simulink model "Experiment_0309_cs_old"  (R2019a)
settings: Solver=ode5  StartTime=0.0  StopTime=6  FixedStep=1/120  RelTol=1e-3
PreLoadFcn:
  | mbxruntime.callbacks.PreLoadFcn(bdroot);
PostLoadFcn:
  | mbxruntime.callbacks.PostLoadFcn(bdroot);
InitFcn:
  | mbxruntime.callbacks.InitFcn(bdroot);
StartFcn:
  | mbxruntime.callbacks.StartFcn(bdroot);
StopFcn:
  | mbxruntime.callbacks.StopFcn(bdroot);
model workspace (MAT data in the model file):
  mbox_table : struct (value not decoded)
  model_closed = 0
  sim_status = 0
undefined symbols (not defined in the file or in its folder): DiscIntNeverNeededParam, InitImageOutputDir, mbxruntime, tabledata
libraries: PreScanSimulinkLibrary x24, simulink_extras x2
(part 1 of 3)
CloseFcn:
  | mbxruntime.callbacks.CloseFcn(bdroot);
settings Model: Creator=PRESCAN  LastModifiedBy=HP
settings DataIOCC: LimitDataPoints=on  SaveFormat=Array  SignalLoggingSaveFormat=ModelDataLogs  ReturnWorkspaceOutputs=off
settings OptimizationCC: ExpressionDepthLimit=2147483647  InitFltsAndDblsToZero=on  LifeSpan=inf
settings DebuggingCC: SaveWithParameterizedLinksMsg=none  UnderspecifiedInitializationDetection=Classic  MergeDetectMultiDrivingBlocksExec=none  SignalResolutionControl=TryResolveAllWithWarning  MultiTaskDSMMsg=warning  MultiTaskCondExecSysMsg=none  FcnCallInpInsideContextMsg=warning  StateNameClashWarn=warning  SFUnexpectedBacktrackingDiag=warning  SFNoUnconditionalDefaultTransitionDiag=warning  SFExecutionAtInitializationDiag=none  ArithmeticOperatorsInVariantConditions=warning
settings HardwareCC: ProdBitPerPointer=32  ProdBitPerSizeT=32  ProdBitPerPtrDiffT=32  ProdLargestAtomicFloat=None  ProdIntDivRoundTo=Undefined  ProdEndianess=Unspecified  ProdWordSize=32  ProdHWDeviceType=32-bit Generic
settings ModelReferenceCC: UpdateModelReferenceTargets=IfOutOfDate  PropagateSignalLabelsOutOfModel=off
settings SFSimCC: SimUseLocalCustomCode=off  SimParseCustomCode=off
settings SFSimCC: SimCustomHeaderCode=|
  | #include "prescan.h"
  | #include "prescan_platform.h"
settings RTWCC: RTWUseLocalCustomCode=off
settings CodeAppCC: StateflowObjectComments=on
settings GRTTargetCC: TargetFcnLib=ansi_tfl_tmw.mat  TargetLangStandard=C89/C90 (ANSI)  GeneratePreprocessorConditionals=Disable all  CombineOutputUpdateFcns=off  GRTInterface=on
settings ConfigComp: CovMetricSettings=dw  CovHtmlReporting=on  CovSaveCumulativeToWorkspaceVar=on  CovSaveSingleToWorkspaceVar=on  CovExternalEMLEnable=off

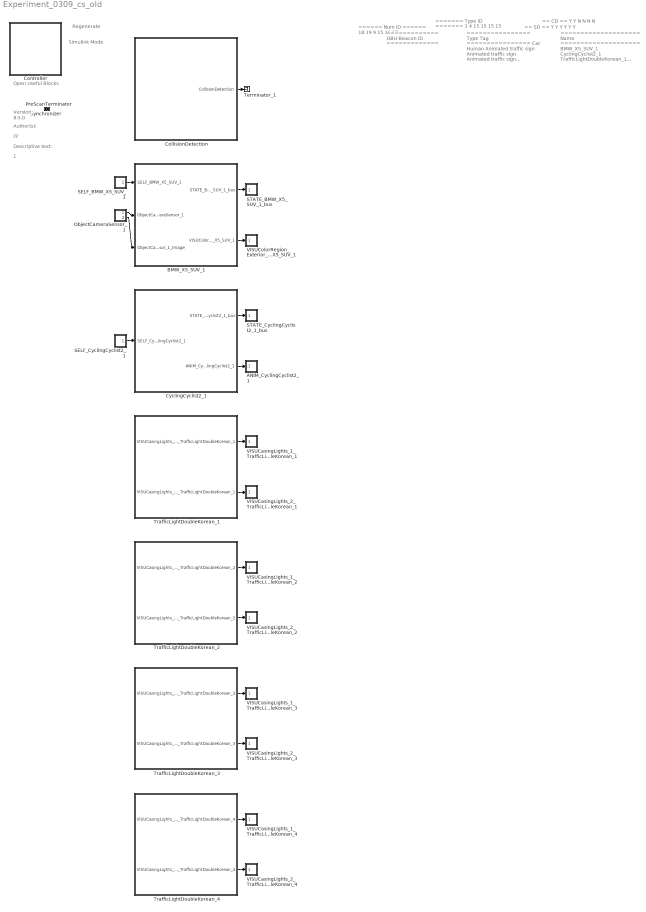
== system Experiment_0309_cs_old ==
  note: Regenerate
  note: Simulink Mode
  note: Open Useful Blocks
  note: 8.5.0
  note: Version:
  note: Author(s):
  note: zz
  note: Descriptive text:
  note: 1
  note: ======
      | Num ID
      | ======
      | 18
      | 19
      | 9
      | 15
      | 16
      | 17
  note: =============
      | OBU-Beacon ID
      | =============
  note: =======
      | Type ID
      | =======
      | 1
      | 4
      | 15
      | 15
      | 15
      | 15
  note: ================
      | Type Tag
      | ================
      | Car
      | Human
      | Animated traffic sign
      | Animated traffic sign
      | Animated traffic sign
      | Animated traffic sign
  note: ==
      | SD
      | ==
      | Y
      | Y
      | Y
      | Y
      | Y
      | Y
  note: ==
      | CD
      | ==
      | Y
      | Y
      | N
      | N
      | N
      | N
  note: ====================
      | Name
      | ====================
      | BMW_X5_SUV_1
      | CyclingCyclist2_1
      | TrafficLightDoubleKorean_1
      | TrafficLightDoubleKorean_2
      | TrafficLightDoubleKorean_3
      | TrafficLightDoubleKorean_4
  ANIM_CyclingCyclist2_1 : Subsystem  Tag=actuator/AnimationOutport  Priority=0  LoadFcn=load('PreScanAnimActuatorData.mat')  mask(PreScan Sink Block: State Animation){}
      mask help: The Cyclist Animation port allows the cyclist to ride the bicycle.
      settings: OpenFcn=open_system([gcb '/Actuator'],'mask')
      mask Help: eval('openHelp(239)')
      mask Display: image(imread('CyclingCyclist2.jpg'))
  BMW_X5_SUV_1 : Subsystem  Tag=WorldObjectSubSystem  InitFcn=UniqueId = '266';
      mask init:
      | modelPath = GenericModelHelper.getGenericModelFilePath('ModelDepo','Vehicles\BMW_X5\BMW_X5.pgmb','cea918691563e9ae3e6a88ec95e6726a');imagePath = GenericModelHelper.getCompilationPicture(modelPath, 'BMW_X5_HighPoly.png');
      mask Display: image(imread(imagePath));color('white');text(0, 0, ' ID=18\n')
  CollisionDetection : Subsystem  Tag=sensor/CollisionDetection  Priority=3  LoadFcn=load('PrescanCollisionDetectionData.mat');load('PrescanCollisionDetectionMessage.mat')  mask(PreScan Source Block: CollisionDetection){}
      mask help: Collision Detection can be used to detect collisions between PreScan components. For Collision Detection the actual component shape is taken into account, so it is not a bounding box approach.
      settings: OpenFcn=open_system([gcb '/Sensor'],'mask')
      mask Help: eval('openHelp(811)')
      mask Display: image(imread('crash.jpg'))
  Controller : Subsystem  Description=44ADF3809AA2EBDEE5B0ED277FCD47A88214DB959FC05F626C23B16B15099040  Priority=-1  LoadFcn=load PreScanControllerData  mask(PreScan Simulation Controller){prescanversion='8.5.0', ModelReferencing=off, TimeStep=3/120, ControlMode=0, PreScanExecutionMode=on, ControllerCount=0, ControllerIndex=0, ControllerOptions=''}
      mask prompts: prescanversion "PreScan Version"; ModelReferencing "Use Model Referencing"; TimeStep "Upload Period [s]"; ControlMode "Control Mode"; PreScanExecutionMode "Execution Mode"; ControllerCount "Controller Count"; ControllerIndex "Controller Index"; ControllerOptions "Controller Options"
      mask help:
      | Please do not remove this block from the compilation sheet,
      | as it connects the model to the PreScan environment.
      mask init:
      | model = bdroot(gcb);
      | ExperimentFile = mbxruntime.findExperimentFile(model,true); %relative path
      | 
      | [d1, d2, d3, prescandata] = prescan_Settings();
      | ModelDepo = fullfile(prescandata,'ModelDepo'); 
      | 
      | RTmode = mbxruntime.getRTMode(model);
      | 
      | SimulationMode = get_param(bdroot,'SimulationMode');
      | if strcmp(SimulationMode, 'rapid-accelerator')
      |     SimulationMode = 'external';
      | end
      | TargetName = get_param(bdroot,'SystemTargetFile');
      settings: ModelCloseFcn=assignin('base',['model_closed_' bdroot],true);
      mask Help: eval('openHelp(812)')
      mask Display: image(imread('prescanlogo.ico'))
  CyclingCyclist2_1 : Subsystem  Tag=WorldObjectSubSystem  InitFcn=UniqueId = '309';
      mask init:
      | imagePath=which('CyclingCyclist2.jpg');
      mask Display: image(imread(imagePath));color('white');text(0, 0, ' ID=19\n')
  ObjectCameraSensor_1 : Subsystem  Tag=sensor/ObjectCamera/data  Priority=3  LoadFcn=load('PrescanOCSData.mat');load('PrescanOCSMessage.mat')  mask(PreScan Source Block: Object Camera Sensor){}
      mask help: The Object Camera Sensor provides information on objects locations.
      settings: OpenFcn=open_system([gcb '/Sensor'],'mask')
      mask Help: eval('openHelp(2401)')
      mask Display: image(imread('ObjectCameraSensorSL.png'))
  PreScanTerminator : Subsystem  Tag=PreScanTerminator  Priority=999  LoadFcn=load PrescanTerminatorData  mask(PreScan Simulation Terminator){TimeStep=3/120}
      mask prompts: TimeStep "Upload Period [s]"
      mask help:
      | Please do not remove this block from the compilation sheet as it
      | connects the model to the PreScan environment.
      mask Help: eval('openHelp(812)')
      mask Display: image(imread('prescanlogo.ico'))
  SELF_BMW_X5_SUV_1 : Subsystem  Tag=sensor/SelfPort  Priority=3  LoadFcn=load('PreScanSelfSensorData.mat')  mask(PreScan Source Block: SELF){}
      mask help:
      | The SELF port shows (state) information of the actor itself. The outputs are position in the experiment's axis system and the GPS coordinates, and the object's absolute velocity and compass heading.
      |
      | For more information, please click Help.
      settings: OpenFcn=open_system([gcb '/Sensor'],'mask')
      mask Help: eval('openHelp(462)')
      mask Display: image(imread('GPS.png'))
  SELF_CyclingCyclist2_1 : Subsystem  Tag=sensor/SelfPort  Priority=3  LoadFcn=load('PreScanSelfSensorData.mat')  mask(PreScan Source Block: SELF){}
      mask help:
      | The SELF port shows (state) information of the actor itself. The outputs are position in the experiment's axis system and the GPS coordinates, and the object's absolute velocity and compass heading.
      |
      | For more information, please click Help.
      settings: OpenFcn=open_system([gcb '/Sensor'],'mask')
      mask Help: eval('openHelp(462)')
      mask Display: image(imread('GPS.png'))
  STATE_BMW_X5_SUV_1_bus : Subsystem  Tag=actuator/StatePort  Priority=0  LoadFcn=load('PreScanStateActuatorData.mat')  mask(PreScan Sink Block: State){}
      mask help:
      | The Actor State contains a vector signal of size (9x1), containing the following signals:
      |
      | -  Position    	(x,y,z)             	[m]
      | -  Velocity    	(vx,vy,vz)         	[m/s]
      | -  Angles       	(Roll, Pitch, Yaw)	[rad]
      |
      | The Actor state is defined in the global axis system.
      | The state is superponed on the Initial position defined in the GUI.
      |
      | For more information, please click Help.
      settings: OpenFcn=open_system([gcb '/Actuator'],'mask')
      mask Help: eval('openHelp(222)')
      mask Display: image(imread('State.png'))
  STATE_CyclingCyclist2_1_bus : Subsystem  Tag=actuator/StatePort  Priority=0  LoadFcn=load('PreScanStateActuatorData.mat')  mask(PreScan Sink Block: State){}
      mask help:
      | The Actor State contains a vector signal of size (9x1), containing the following signals:
      |
      | -  Position    	(x,y,z)             	[m]
      | -  Velocity    	(vx,vy,vz)         	[m/s]
      | -  Angles       	(Roll, Pitch, Yaw)	[rad]
      |
      | The Actor state is defined in the global axis system.
      | The state is superponed on the Initial position defined in the GUI.
      |
      | For more information, please click Help.
      settings: OpenFcn=open_system([gcb '/Actuator'],'mask')
      mask Help: eval('openHelp(222)')
      mask Display: image(imread('State.png'))
  Synchronizer : Subsystem  Tag=PreScanSynchronizer  Priority=1  LoadFcn=load PrescanSynchronizeData  mask(PreScan Simulation Core Block){TimeStep=3/120}
      mask prompts: TimeStep "Timestep [s]"
      mask help:
      | Please do not remove this block from the PreScan compilation sheet,
      | as it contains essential configuration parameters for a PreScan simulation.
      settings: DeleteFcn=PreScanBlockDeleteFcn;
      mask Display: image(imread('prescanlogo.ico'))
  Terminator_1 : Terminator
  TrafficLightDoubleKorean_1 : Subsystem  Tag=WorldObjectSubSystem  InitFcn=UniqueId = '262';
      mask init:
      | imagePath=which('TrafficLightDoubleKorean.jpg');
      mask Display: image(imread(imagePath));color('white');text(0, 0, ' ID=9\n')
  TrafficLightDoubleKorean_2 : Subsystem  Tag=WorldObjectSubSystem  InitFcn=UniqueId = '263';
      mask init:
      | imagePath=which('TrafficLightDoubleKorean.jpg');
      mask Display: image(imread(imagePath));color('white');text(0, 0, ' ID=15\n')
  TrafficLightDoubleKorean_3 : Subsystem  Tag=WorldObjectSubSystem  InitFcn=UniqueId = '264';
      mask init:
      | imagePath=which('TrafficLightDoubleKorean.jpg');
      mask Display: image(imread(imagePath));color('white');text(0, 0, ' ID=16\n')
  TrafficLightDoubleKorean_4 : Subsystem  Tag=WorldObjectSubSystem  InitFcn=UniqueId = '265';
      mask init:
      | imagePath=which('TrafficLightDoubleKorean.jpg');
      mask Display: image(imread(imagePath));color('white');text(0, 0, ' ID=17\n')
  VISUCasingLights_1_TrafficLightDoubleKorean_1 : Subsystem  Tag=actuator/VisuCasingLights  Priority=0  mask(PreScan Sink Block: VisuTrafficLight){UniqueID=262, ColorsObjectQuery=, Colors=[]}
      mask prompts: UniqueID "Parent Unique Identifier"; ColorsObjectQuery "Query for Color Object"; Colors "Matrix of colors"
      mask help:
      | The VisuTrafficLight block provides a way to animate traffic lights: switch on and off individual lights.
      |
      | For more information, please click Help.
      settings: OpenFcn=open_system([gcb '/Actuator'],'mask')
      mask Help: eval('openHelp(731)')
      mask Display: image(imread('TrafficLightCasing.png'))
  VISUCasingLights_1_TrafficLightDoubleKorean_2 : Subsystem  Tag=actuator/VisuCasingLights  Priority=0  mask(PreScan Sink Block: VisuTrafficLight){UniqueID=263, ColorsObjectQuery=, Colors=[]}
      mask prompts: UniqueID "Parent Unique Identifier"; ColorsObjectQuery "Query for Color Object"; Colors "Matrix of colors"
      mask help:
      | The VisuTrafficLight block provides a way to animate traffic lights: switch on and off individual lights.
      |
      | For more information, please click Help.
      settings: OpenFcn=open_system([gcb '/Actuator'],'mask')
      mask Help: eval('openHelp(731)')
      mask Display: image(imread('TrafficLightCasing.png'))
  VISUCasingLights_1_TrafficLightDoubleKorean_3 : Subsystem  Tag=actuator/VisuCasingLights  Priority=0  mask(PreScan Sink Block: VisuTrafficLight){UniqueID=264, ColorsObjectQuery=, Colors=[]}
      mask prompts: UniqueID "Parent Unique Identifier"; ColorsObjectQuery "Query for Color Object"; Colors "Matrix of colors"
      mask help:
      | The VisuTrafficLight block provides a way to animate traffic lights: switch on and off individual lights.
      |
      | For more information, please click Help.
      settings: OpenFcn=open_system([gcb '/Actuator'],'mask')
      mask Help: eval('openHelp(731)')
      mask Display: image(imread('TrafficLightCasing.png'))
  VISUCasingLights_1_TrafficLightDoubleKorean_4 : Subsystem  Tag=actuator/VisuCasingLights  Priority=0  mask(PreScan Sink Block: VisuTrafficLight){UniqueID=265, ColorsObjectQuery=, Colors=[]}
      mask prompts: UniqueID "Parent Unique Identifier"; ColorsObjectQuery "Query for Color Object"; Colors "Matrix of colors"
      mask help:
      | The VisuTrafficLight block provides a way to animate traffic lights: switch on and off individual lights.
      |
      | For more information, please click Help.
      settings: OpenFcn=open_system([gcb '/Actuator'],'mask')
      mask Help: eval('openHelp(731)')
      mask Display: image(imread('TrafficLightCasing.png'))
  VISUCasingLights_2_TrafficLightDoubleKorean_1 : Subsystem  Tag=actuator/VisuCasingLights  Priority=0  mask(PreScan Sink Block: VisuTrafficLight){UniqueID=262, ColorsObjectQuery=, Colors=[]}
      mask prompts: UniqueID "Parent Unique Identifier"; ColorsObjectQuery "Query for Color Object"; Colors "Matrix of colors"
      mask help:
      | The VisuTrafficLight block provides a way to animate traffic lights: switch on and off individual lights.
      |
      | For more information, please click Help.
      settings: OpenFcn=open_system([gcb '/Actuator'],'mask')
      mask Help: eval('openHelp(731)')
      mask Display: image(imread('TrafficLightCasing.png'))
  VISUCasingLights_2_TrafficLightDoubleKorean_2 : Subsystem  Tag=actuator/VisuCasingLights  Priority=0  mask(PreScan Sink Block: VisuTrafficLight){UniqueID=263, ColorsObjectQuery=, Colors=[]}
      mask prompts: UniqueID "Parent Unique Identifier"; ColorsObjectQuery "Query for Color Object"; Colors "Matrix of colors"
      mask help:
      | The VisuTrafficLight block provides a way to animate traffic lights: switch on and off individual lights.
      |
      | For more information, please click Help.
      settings: OpenFcn=open_system([gcb '/Actuator'],'mask')
      mask Help: eval('openHelp(731)')
      mask Display: image(imread('TrafficLightCasing.png'))
  VISUCasingLights_2_TrafficLightDoubleKorean_3 : Subsystem  Tag=actuator/VisuCasingLights  Priority=0  mask(PreScan Sink Block: VisuTrafficLight){UniqueID=264, ColorsObjectQuery=, Colors=[]}
      mask prompts: UniqueID "Parent Unique Identifier"; ColorsObjectQuery "Query for Color Object"; Colors "Matrix of colors"
      mask help:
      | The VisuTrafficLight block provides a way to animate traffic lights: switch on and off individual lights.
      |
      | For more information, please click Help.
      settings: OpenFcn=open_system([gcb '/Actuator'],'mask')
      mask Help: eval('openHelp(731)')
      mask Display: image(imread('TrafficLightCasing.png'))
  VISUCasingLights_2_TrafficLightDoubleKorean_4 : Subsystem  Tag=actuator/VisuCasingLights  Priority=0  mask(PreScan Sink Block: VisuTrafficLight){UniqueID=265, ColorsObjectQuery=, Colors=[]}
      mask prompts: UniqueID "Parent Unique Identifier"; ColorsObjectQuery "Query for Color Object"; Colors "Matrix of colors"
      mask help:
      | The VisuTrafficLight block provides a way to animate traffic lights: switch on and off individual lights.
      |
      | For more information, please click Help.
      settings: OpenFcn=open_system([gcb '/Actuator'],'mask')
      mask Help: eval('openHelp(731)')
      mask Display: image(imread('TrafficLightCasing.png'))
  VISUColorRegion_Exterior_BMW_X5_SUV_1 : Subsystem  Tag=actuator/ColorRegion  Priority=0  LoadFcn=load('PrescanColorData')  mask(PreScan Sink Block: VisuTextureColor){}
      mask help:
      | The VisuTextureColor block provides a way to adapt the color of a vehicle.
      |
      | For more information, please click Help.
      settings: OpenFcn=open_system([gcb '/Actuator'],'mask')
      mask Help: eval('openHelp(230)')
      mask Display: image(imread('TextureColor.png'))
  wires:
  BMW_X5_SUV_1/1(STATE_BMW_X5_SUV_1_bus) -> STATE_BMW_X5_SUV_1_bus/1(STATE_BMW_X5_SUV_1_bus)
  SELF_BMW_X5_SUV_1/1(SELF_BMW_X5_SUV_1) -> BMW_X5_SUV_1/1(SELF_BMW_X5_SUV_1)
  ObjectCameraSensor_1/1(ObjectCameraSensor_1) -> BMW_X5_SUV_1/2(ObjectCameraSensor_1)
  ObjectCameraSensor_1/2(ObjectCameraSensor_1_Image) -> BMW_X5_SUV_1/3(ObjectCameraSensor_1_Image)
  BMW_X5_SUV_1/2(VISUColorRegion_Exterior_BMW_X5_SUV_1) -> VISUColorRegion_Exterior_BMW_X5_SUV_1/1(VISUColorRegion_Exterior_BMW_X5_SUV_1)
  CyclingCyclist2_1/1(STATE_CyclingCyclist2_1_bus) -> STATE_CyclingCyclist2_1_bus/1(STATE_CyclingCyclist2_1_bus)
  CyclingCyclist2_1/2(ANIM_CyclingCyclist2_1) -> ANIM_CyclingCyclist2_1/1(ANIM_CyclingCyclist2_1)
  SELF_CyclingCyclist2_1/1(SELF_CyclingCyclist2_1) -> CyclingCyclist2_1/1(SELF_CyclingCyclist2_1)
  TrafficLightDoubleKorean_1/1(VISUCasingLights_1_TrafficLightDoubleKorean_1) -> VISUCasingLights_1_TrafficLightDoubleKorean_1/1(VISUCasingLights_1_TrafficLightDoubleKorean_1)
  TrafficLightDoubleKorean_1/2(VISUCasingLights_2_TrafficLightDoubleKorean_1) -> VISUCasingLights_2_TrafficLightDoubleKorean_1/1(VISUCasingLights_2_TrafficLightDoubleKorean_1)
  TrafficLightDoubleKorean_2/1(VISUCasingLights_1_TrafficLightDoubleKorean_2) -> VISUCasingLights_1_TrafficLightDoubleKorean_2/1(VISUCasingLights_1_TrafficLightDoubleKorean_2)
  TrafficLightDoubleKorean_2/2(VISUCasingLights_2_TrafficLightDoubleKorean_2) -> VISUCasingLights_2_TrafficLightDoubleKorean_2/1(VISUCasingLights_2_TrafficLightDoubleKorean_2)
  TrafficLightDoubleKorean_3/1(VISUCasingLights_1_TrafficLightDoubleKorean_3) -> VISUCasingLights_1_TrafficLightDoubleKorean_3/1(VISUCasingLights_1_TrafficLightDoubleKorean_3)
  TrafficLightDoubleKorean_3/2(VISUCasingLights_2_TrafficLightDoubleKorean_3) -> VISUCasingLights_2_TrafficLightDoubleKorean_3/1(VISUCasingLights_2_TrafficLightDoubleKorean_3)
  TrafficLightDoubleKorean_4/1(VISUCasingLights_1_TrafficLightDoubleKorean_4) -> VISUCasingLights_1_TrafficLightDoubleKorean_4/1(VISUCasingLights_1_TrafficLightDoubleKorean_4)
  TrafficLightDoubleKorean_4/2(VISUCasingLights_2_TrafficLightDoubleKorean_4) -> VISUCasingLights_2_TrafficLightDoubleKorean_4/1(VISUCasingLights_2_TrafficLightDoubleKorean_4)
  CollisionDetection/1(CollisionDetection) -> Terminator_1/1

== system Experiment_0309_cs_old/ANIM_CyclingCyclist2_1 ==
  ANIM_CyclingCyclist2_1 : Inport  Tag=inport/AnimationOutport  OutDataTypeStr=Bus: PRESCAN_ANIMACTUATORDATA  PortDimensions=2  SampleTime=3/120  BusOutputAsStruct=on
  Actuator : S-Function  FunctionName=sfun_CyclistAnimActuator  Parameters=UniqueID, uint8([ParentObject 0]), TimeStep  SFunctionDeploymentMode=off  EnableBusSupport=off  mask(PreScan Sink Block: State Animation){UniqueID=309, ParentObject=CyclingCyclist2_1, TimeStep=3/120}
      mask prompts: UniqueID "Auto-Assigned: Unique ID"; ParentObject "Auto-Assigned: ParentObject"; TimeStep "Auto-Assigned: Upload Period [s]"
      mask help: The Cyclist Animation port allows the cyclist to ride the bicycle.
      mask Help: eval('openHelp(239)')
      mask Display: image(imread('CyclingCyclist2.jpg'))
  wires:
  ANIM_CyclingCyclist2_1/1 -> Actuator/1

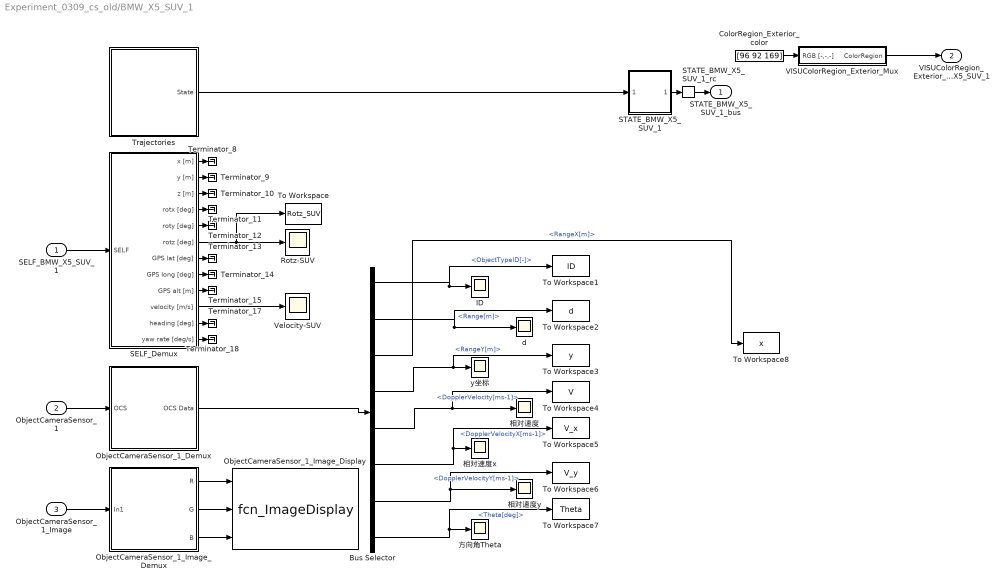
== system Experiment_0309_cs_old/BMW_X5_SUV_1 ==
  SELF_BMW_X5_SUV_1 : Inport  Tag=inport/SelfPort  OutDataTypeStr=Bus: PRESCAN_SELFSENSORDATA  PortDimensions=1  SampleTime=3/120  BusOutputAsStruct=on
  ObjectCameraSensor_1 : Inport  Tag=inport/ObjectCamera/data  Port=2  OutDataTypeStr=Bus: PRESCAN_OCS_MESSAGE  PortDimensions=7  SampleTime=1/40  BusOutputAsStruct=on
  ObjectCameraSensor_1_Image : Inport  Tag=inport/ObjectCamera/image  Port=3  OutDataTypeStr=uint8  SampleTime=1/40  BusOutputAsStruct=on
  Bus Selector : BusSelector  OutputSignals=ObjectTypeID[-],Range[m],RangeX[m],RangeY[m],DopplerVelocity[ms-1],DopplerVelocityX[ms-1],DopplerVelocityY[ms-1],Theta[deg]
  ColorRegion_Exterior_color : Constant  Tag=VisuLightConst  Value=[96 92 169]
  ID : Scope
  ObjectCameraSensor_1_Demux : Subsystem  Tag=demux/OCS  mask(PreScan Demux Block: Object Camera Sensor){detectableObjects=7}
      mask prompts: detectableObjects "Max. detectable objects"
      settings: DeleteFcn=PreScanBlockDeleteFcn;
      mask Help: eval('openHelp(2401)')
      mask Display:
      | port_label('input', 1, 'OCS')
      | port_label('output', 1, 'OCS Data')
  ObjectCameraSensor_1_Image_Demux : Subsystem  Tag=demux/Camera/Color  mask{SensorName=ObjectCameraSensor_1, hres=320, vres=240}
      mask prompts: SensorName "Sensor Name"; hres "Horizontal Resolution"; vres "Vertical Resolution"
      mask Help: eval('openHelp(2401)')
      mask Display:
      | fprintf('MONO CAMERA:\n Color\n %s \n %d x %d px',SensorName,hres,vres)
      | port_label('output',1,'R')
      | port_label('output',2,'G')
      | port_label('output',3,'B')
  ObjectCameraSensor_1_Image_Display : M-S-Function  Tag=CameraSensor_Color_Display  InitFcn=InitImageOutputDir(gcb);  FunctionName=fcn_ImageDisplay  Parameters=SensorName EnableDisplay EnablePosition DisplayPosition FigureHandle SaveResults BitmapFormat TempOutputDir CameraType DataType  mask(PreScan Color Display Block){SensorName=ObjectCameraSensor_1_Image, EnableDisplay=on, EnablePosition=off, DisplayPosition=[10 10 320 240], FigureHandle=26601, SaveResults=off, Format=PNG, TempOutputDir=0, CameraType=Mono, DataType=uint8}
      mask prompts: SensorName "User Specified: Title of Display"; EnableDisplay "Active"; EnablePosition "Set Display window position"; DisplayPosition "Display window position [xpos ypos width height]"; FigureHandle "Unique Handle"; SaveResults "Save results"; TempOutputDir "OutputDir"; CameraType "Camera Type"; DataType "Image Data Type"
      mask help: This block displays the RGB output of a PreScan camera sensor.
      mask init:
      | if EnableDisplay
      |     EnableString='';
      |     EnableColor='gray';
      | else
      |     EnableString='INACTIVE';
      |     EnableColor='red';
      | end
      | switch Format
      |     case 1
      |         BitmapFormat = 'png';
      |     case 2
      |         BitmapFormat = 'bmp';
      |     case 3
      |         BitmapFormat = 'jpg';
      | end 
      | if CameraType==1
      |     CameraTypeName='MONO';
      |     PortNumber=0;
      | else
      |     CameraTypeName='STEREO';
      |     PortNumber=3;
      | end
      settings: CopyFcn=CopyFcnDisplay  DeleteFcn=PreScanBlockDeleteFcn;  ModelCloseFcn=fcn_ImageDisplay_ModelCloseFcn
      mask Help: eval('openHelp(2401)')
      mask Callback EnablePosition:
      | MV=get_param(gcb,'MaskVisibilities');
      | if strcmp(get_param(gcb,'EnablePosition'),'on')
      |     MV{4}='on';
      | else
      |     MV{4}='off';
      | end
      | set_param(gcb,'MaskVisibilities',MV);
      | clear MV;
      mask TypeOptions Format: PNG | BMP | JPG
      mask TypeOptions CameraType: Mono | Stereo
      mask TypeOptions DataType: uint8 | single
      mask Display:
      | color(EnableColor);
      | fprintf('%s\n DISPLAY:\n Color \n %s',EnableString,SensorName)
      | port_label('input',1,'R')
      | port_label('input',2,'G')
      | port_label('input',3,'B')
      | port_label('input',PortNumber+1,'R')
      | port_label('input',PortNumber+2,'G')
      | port_label('input',PortNumber+3,'B')
  Rotz-SUV : Scope
  SELF_Demux : Subsystem  Tag=demux/SelfPort  mask(PreScan Demux Block:){}
      mask help:
      | The SELF port shows (state) information of the actor itself. The outputs are position in the experiment's axis system and the GPS coordinates, and the object's absolute velocity and compass heading.
      |
      | For more information, please click Help.
      settings: DeleteFcn=PreScanBlockDeleteFcn;
      mask Help: eval('openHelp(462)')
      mask Display:
      | port_label('output',1,'x [m]')
      | port_label('output',2,'y [m]')
      | port_label('output',3,'z [m]','texmode','on')
      | port_label('output',4,'Rotx [deg]','texmode','on')
      | port_label('output',5,'Roty [deg]','texmode','on')
      | port_label('output',6,'Rotz [deg]','texmode','on')
      | port_label('output',7,'GPS lat [deg]','texmode','on')
      | port_label('output',8,'GPS long [deg]','texmode','on')
      | port_label('output',9,'GPS alt [m]','texmode','on')
      | port_label('output',10,'Velocity [m/s]')
      | port_label('output',11,'Heading [deg]')
      | port_label('output',12,'Yaw rate [deg/s]')
  STATE_BMW_X5_SUV_1 : Subsystem  Tag=mux/StatePort  Priority=0  LoadFcn=load PrescanStateActuatorData  mask(PreScan Sink Block: State){x0=52.8761, y0=6.1543, z0=0.69, Roll0=0, Pitch0=0, Yaw0=90, TimeStep=3/120}
      mask prompts: x0 "Ini x-position VEHICLE wrt GLOBAL axis system [m]"; y0 "Ini y-position VEHICLE wrt GLOBAL axis system [m]"; z0 "Ini z-position VEHICLE wrt GLOBAL axis system [m]"; Roll0 "Ini roll-angle BODY wrt VEHICLE axis system [deg]"; Pitch0 "Ini pitch-angle BODY wrt VEHICLE axis system [deg]"; Yaw0 "Ini yaw-angle VEHICLE wrt GLOBAL axis system [deg]"; TimeStep "Auto-Assigned: Upload Period [s]"
      mask help:
      | The Actor State contains a vector signal of size (9x1), containing the following signals:
      |
      | -  Position                  (x,y,z)                                     [m]
      | -  Velocity                  (vx,vy,vz)                               [m/s]
      | -  Angles                    (Roll, Pitch, Yaw)                   [rad]
      |
      | The Actor state is defined in the global axis system.
      | The state is superponed on the Initial position defined in the GUI.
      |
      | For more information, please click Help.
      settings: DeleteFcn=PreScanBlockDeleteFcn;
      mask Help: eval('openHelp(222)')
      mask Display: image(imread('State.png'))
  STATE_BMW_X5_SUV_1_rc : RateTransition  Tag=mux_rc/StatePort  OutPortSampleTimeOpt=Inherit
  Terminator_{8..15,17..18} (10 alike) : Terminator
  To Workspace : ToWorkspace  VariableName=Rotz_SUV  SaveFormat=Timeseries  SampleTime=-1
  To Workspace1 : ToWorkspace  VariableName=ID  SaveFormat=Timeseries  SampleTime=-1
  To Workspace2 : ToWorkspace  VariableName=d  SaveFormat=Timeseries  SampleTime=-1
  To Workspace3 : ToWorkspace  VariableName=y  SaveFormat=Timeseries  SampleTime=-1
  To Workspace4 : ToWorkspace  VariableName=V  SaveFormat=Timeseries  SampleTime=-1
  To Workspace5 : ToWorkspace  VariableName=V_x  SaveFormat=Timeseries  SampleTime=-1
  To Workspace6 : ToWorkspace  VariableName=V_y  SaveFormat=Timeseries  SampleTime=-1
  To Workspace7 : ToWorkspace  VariableName=Theta  SaveFormat=Timeseries  SampleTime=-1
  To Workspace8 : ToWorkspace  VariableName=x  SaveFormat=Timeseries  SampleTime=-1
  Trajectories : Subsystem  Tag=Trajectories  mask(PreScan Source Block: Trajectories){}
      mask help:
      | The Trajectory block contains the trajectories defined in the PreScan Experiment Editor. The output of the trajectory block is the (vehicle) State.
      |
      | For more information, please click Help.
      settings: DeleteFcn=PreScanBlockDeleteFcn;
      mask Help: eval('openHelp(312)')
      mask Display: image(imread('Trajectory.png'));
  VISUColorRegion_Exterior_Mux : Subsystem  Tag=mux/MuxColorRegion  LoadFcn=load PrescanColorData  mask(PreScan User Interface: VisuTextureColor){}
      mask help:
      | The VisuTextureColor block provides a way to adapt the color of a vehicle.
      |
      | For more information, please click Help.
      settings: DeleteFcn=PreScanBlockDeleteFcn;
      mask Help: eval('openHelp(230)')
  Velocity-SUV : Scope
  d : Scope
  y坐标 : Scope
  方向角Theta : Scope
  相对速度 : Scope
  相对速度x : Scope
  相对速度y : Scope
  STATE_BMW_X5_SUV_1_bus : Outport  Tag=outport/StatePort  OutDataTypeStr=Bus: PRESCAN_STATEACTUATORDATA  PortDimensions=1  SampleTime=3/120
  VISUColorRegion_Exterior_BMW_X5_SUV_1 : Outport  Tag=outport/ColorRegion  Port=2  OutDataTypeStr=Bus: PRESCAN_COLOR_DATA  PortDimensions=1  SampleTime=3/120
  wires:
  ObjectCameraSensor_1_Demux/1(OCS Data) -> Bus Selector/1
  SELF_Demux/6(rotz [deg]) -> To Workspace/1, Rotz-SUV/1
  STATE_BMW_X5_SUV_1_rc/1 -> STATE_BMW_X5_SUV_1_bus/1
  STATE_BMW_X5_SUV_1/1(StateBus) -> STATE_BMW_X5_SUV_1_rc/1
  SELF_BMW_X5_SUV_1/1 -> SELF_Demux/1(SELF)
  ObjectCameraSensor_1/1 -> ObjectCameraSensor_1_Demux/1(OCS)
  ObjectCameraSensor_1_Image/1 -> ObjectCameraSensor_1_Image_Demux/1(In1)
  ObjectCameraSensor_1_Image_Demux/1(R) -> ObjectCameraSensor_1_Image_Display/1
  ObjectCameraSensor_1_Image_Demux/2(G) -> ObjectCameraSensor_1_Image_Display/2
  ObjectCameraSensor_1_Image_Demux/3(B) -> ObjectCameraSensor_1_Image_Display/3
  VISUColorRegion_Exterior_Mux/1(ColorRegion) -> VISUColorRegion_Exterior_BMW_X5_SUV_1/1
  ColorRegion_Exterior_color/1 -> VISUColorRegion_Exterior_Mux/1(RGB [-,-,-])
  Trajectories/1(State) -> STATE_BMW_X5_SUV_1/1(State)
  Bus Selector/1 -> To Workspace1/1, ID/1  "<ObjectTypeID[-]>"
  Bus Selector/2 -> d/1, To Workspace2/1  "<Range[m]>"
  Bus Selector/5 -> To Workspace4/1, 相对速度/1  "<DopplerVelocity[ms-1]>"
  Bus Selector/6 -> To Workspace5/1, 相对速度x/1  "<DopplerVelocityX[ms-1]>"
  Bus Selector/7 -> To Workspace6/1, 相对速度y/1  "<DopplerVelocityY[ms-1]>"
  Bus Selector/8 -> To Workspace7/1, 方向角Theta/1  "<Theta[deg]>"
  SELF_Demux/1(x [m]) -> Terminator_8/1
  SELF_Demux/2(y [m]) -> Terminator_9/1
  SELF_Demux/3(z [m]) -> Terminator_10/1
  SELF_Demux/4(rotx [deg]) -> Terminator_11/1
  SELF_Demux/5(roty [deg]) -> Terminator_12/1
  SELF_Demux/7(GPS lat [deg]) -> Terminator_13/1
  SELF_Demux/8(GPS long [deg]) -> Terminator_14/1
  SELF_Demux/9(GPS alt [m]) -> Terminator_15/1
  SELF_Demux/10(velocity [m/s]) -> Velocity-SUV/1
  SELF_Demux/11(heading [deg]) -> Terminator_17/1
  SELF_Demux/12(yaw rate [deg/s]) -> Terminator_18/1
  Bus Selector/4 -> To Workspace3/1, y坐标/1  "<RangeY[m]>"
  Bus Selector/3 -> To Workspace8/1  "<RangeX[m]>"

== system Experiment_0309_cs_old/CollisionDetection ==
  Sensor : S-Function  FunctionName=sfun_CollisionDetection  Parameters=detectableCollisions, timestep  SFunctionDeploymentMode=off  EnableBusSupport=off  mask(PreScan Source Block: CollisionDetection){detectableCollisions=5, timestep=3/120}
      mask prompts: detectableCollisions "Max detectable collisions:"; timestep "MATLAB timestep:"
      mask help: Collision Detection can be used to detect collisions between PreScan components. For Collision Detection the actual component shape is taken into account, so it is not a bounding box approach.
      mask Help: eval('openHelp(811)')
      mask Display: image(imread('crash.jpg'))
  CollisionDetection : Outport  Tag=outport/CollisionDetection  OutDataTypeStr=Bus: PRESCAN_COLLISIONDETECTION_MESSAGE  PortDimensions=5  SampleTime=3/120
  wires:
  Sensor/1 -> CollisionDetection/1

== system Experiment_0309_cs_old/Controller ==
  Terminator : Terminator
  sfun_Controller : S-Function  FunctionName=sfun_Controller  Parameters=SParameter1, SParameter2, SParameter3, SParameter4, SParameter5, SParameter6, SParameter7, SParameter8, SParameter9, SParameter10, SampleTime  SFunctionDeploymentMode=off  EnableBusSupport=off  mask(Legacy Function){SFunctionSpec=void prescan_outputFcn(void** work1, PRESCAN_CONTROLLERDATA y1[1]), SParameter1=uint8([ExperimentFile 0]), SParameter2=uint8([ModelDepo 0]), SParameter3=uint8([ControllerOptions 0]), SParameter4=RTmode, SParameter5=PreScanExecutionMode, SParameter6=ControlMode, SParameter7=ControllerCount, SParameter8=ControllerIndex, SParameter9=uint8([SimulationMode 0]), SParameter10=uint8([TargetName 0]), SampleTime=TimeStep, ShowSpec=on}
      mask prompts: SParameter1 "P1:"; SParameter2 "P2:"; SParameter3 "P3:"; SParameter4 "P4:"; SParameter5 "P5:"; SParameter6 "P6:"; SParameter7 "P7:"; SParameter8 "P8:"; SParameter9 "P9:"; SParameter10 "P10:"; SampleTime "Sample time (-1 for inherited):"; ShowSpec "Display function specification"
      mask help:
      | This block allows you to call the legacy functions specified by the following Legacy Code Tool definition:
      | def.SFunctionName = 'sfun_Controller';
      | def.OutputFcnSpec = 'void prescan_outputFcn(void** work1, PRESCAN_CONTROLLERDATA y1[1])';
      | def.StartFcnSpec = 'void prescan_startFcn(void ** work1, uint8 p1[], uint8 p2[], uint8 p3[], double p4, double p5, double p6, double p7, double p8, uint8 p9[], uint8 p10[])';
      | def.TerminateFcnSpec = 'void prescan_terminateFcn(void** work1)';
      | def.HeaderFiles = {'prescan_controller_data.h', 'prescan_SFunLibrary.h', 'prescan_CreateLogHandler.h', 'prescan_CreateErrorHandler.h', 'prescan_modify.h', 'ModuleDLL.h'};
      | def.SourceFiles = {'prescan_MexLogHandler.c', 'prescan_SimStructErrorHandler.c', 'prescan_LogHandler.c', 'prescan_ErrorHandler.c', 'prescan_Modify.c'};
      | def.HostLibFiles = {'sensorinterfaced.lib'};
      | def.TargetLibFiles = {'sensorinterfaced.so'};
      | def.IncPaths = {'.', 'C:\projects\prescan\rt_vislibrary\vis\..\pimp\include\sensors\InterfaceRTW'};
      | def.SrcPaths = {'C:\projects\prescan\rt_vislibrary\vis\..\pimp\include\sensors\InterfaceRTW', 'C:\projects\prescan\rt_vislibrary\vis\..\pimp\include\sensors\InterfaceRTW\ccurrt'};
      | def.LibPaths = {'C:\\projects\\prescan\\vislibrary_build\lib'};
      | def.SampleTime = 'parameterized';
      mask Help: <p>This block was generated automatically by the Legacy Code Tool. For detailed help on this tool, call<a href="matlab:legacy_code('help')"> legacy_code('help')</a>.</p>
      mask Callback ShowSpec:
      | if strcmp(get_param(gcbh, 'ShowSpec'), 'on')
      |   set_param(gcbh, 'MaskDisplay', sprintf('fprintf(''%s'');', get_param(gcbh, 'SFunctionSpec')));
      | else
      |   set_param(gcbh, 'MaskDisplay', sprintf('fprintf(''%s'');', get_param(gcbh, 'FunctionName')));
      | end
      mask Display: fprintf('void prescan_outputFcn(void** work1, PRESCAN_CONTROLLERDATA y1[1])');
  wires:
  sfun_Controller/1 -> Terminator/1

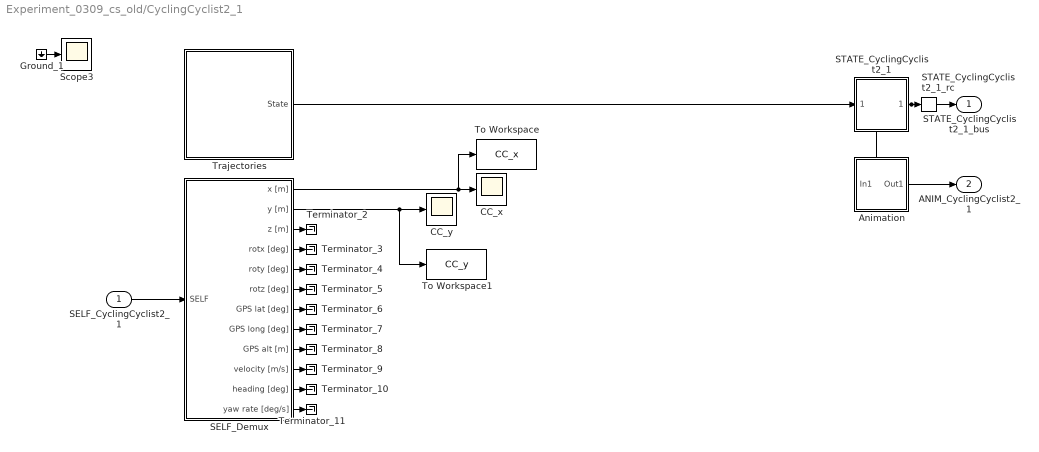
== system Experiment_0309_cs_old/CyclingCyclist2_1 ==
  SELF_CyclingCyclist2_1 : Inport  Tag=inport/SelfPort  OutDataTypeStr=Bus: PRESCAN_SELFSENSORDATA  PortDimensions=1  SampleTime=3/120  BusOutputAsStruct=on
  Animation : Subsystem  Tag=CyclistAnimation  mask(Prescan Conversion Block: Cyclist Animation){TimeStep=3/120}
      mask prompts: TimeStep "Auto-Assigned: Upload Period [s]"
      mask help: The Cyclist animation block converts the State signal into the animation signal for proper animation of the cycling cyclist.
      mask Help: eval('openHelp(239)');
      mask Display: image(imread('CyclingCyclist2.jpg'));
  CC_x : Scope
  CC_y : Scope
  Ground_1 : Ground
  SELF_Demux : Subsystem  Tag=demux/SelfPort  mask(PreScan Demux Block:){}
      mask help:
      | The SELF port shows (state) information of the actor itself. The outputs are position in the experiment's axis system and the GPS coordinates, and the object's absolute velocity and compass heading.
      |
      | For more information, please click Help.
      settings: DeleteFcn=PreScanBlockDeleteFcn;
      mask Help: eval('openHelp(462)')
      mask Display:
      | port_label('output',1,'x [m]')
      | port_label('output',2,'y [m]')
      | port_label('output',3,'z [m]','texmode','on')
      | port_label('output',4,'Rotx [deg]','texmode','on')
      | port_label('output',5,'Roty [deg]','texmode','on')
      | port_label('output',6,'Rotz [deg]','texmode','on')
      | port_label('output',7,'GPS lat [deg]','texmode','on')
      | port_label('output',8,'GPS long [deg]','texmode','on')
      | port_label('output',9,'GPS alt [m]','texmode','on')
      | port_label('output',10,'Velocity [m/s]')
      | port_label('output',11,'Heading [deg]')
      | port_label('output',12,'Yaw rate [deg/s]')
  STATE_CyclingCyclist2_1 : Subsystem  Tag=mux/StatePort  Priority=0  LoadFcn=load PrescanStateActuatorData  mask(PreScan Sink Block: State){x0=56.1734, y0=31.2023, z0=0, Roll0=0, Pitch0=0, Yaw0=89.2836, TimeStep=3/120}
      mask prompts: x0 "Ini x-position VEHICLE wrt GLOBAL axis system [m]"; y0 "Ini y-position VEHICLE wrt GLOBAL axis system [m]"; z0 "Ini z-position VEHICLE wrt GLOBAL axis system [m]"; Roll0 "Ini roll-angle BODY wrt VEHICLE axis system [deg]"; Pitch0 "Ini pitch-angle BODY wrt VEHICLE axis system [deg]"; Yaw0 "Ini yaw-angle VEHICLE wrt GLOBAL axis system [deg]"; TimeStep "Auto-Assigned: Upload Period [s]"
      mask help:
      | The Actor State contains a vector signal of size (9x1), containing the following signals:
      |
      | -  Position                  (x,y,z)                                     [m]
      | -  Velocity                  (vx,vy,vz)                               [m/s]
      | -  Angles                    (Roll, Pitch, Yaw)                   [rad]
      |
      | The Actor state is defined in the global axis system.
      | The state is superponed on the Initial position defined in the GUI.
      |
      | For more information, please click Help.
      settings: DeleteFcn=PreScanBlockDeleteFcn;
      mask Help: eval('openHelp(222)')
      mask Display: image(imread('State.png'))
  STATE_CyclingCyclist2_1_rc : RateTransition  Tag=mux_rc/StatePort  OutPortSampleTimeOpt=Inherit
  Scope3 : Scope
  Terminator_{2..11} (10 alike) : Terminator
  To Workspace : ToWorkspace  VariableName=CC_x  SaveFormat=Timeseries  SampleTime=-1
  To Workspace1 : ToWorkspace  VariableName=CC_y  SaveFormat=Timeseries  SampleTime=-1
  Trajectories : Subsystem  Tag=Trajectories  mask(PreScan Source Block: Trajectories){}
      mask help:
      | The Trajectory block contains the trajectories defined in the PreScan Experiment Editor. The output of the trajectory block is the (vehicle) State.
      |
      | For more information, please click Help.
      settings: DeleteFcn=PreScanBlockDeleteFcn;
      mask Help: eval('openHelp(312)')
      mask Display: image(imread('Trajectory.png'));
  STATE_CyclingCyclist2_1_bus : Outport  Tag=outport/StatePort  OutDataTypeStr=Bus: PRESCAN_STATEACTUATORDATA  PortDimensions=1  SampleTime=3/120
  ANIM_CyclingCyclist2_1 : Outport  Tag=outport/AnimationOutport  Port=2  OutDataTypeStr=Bus: PRESCAN_ANIMACTUATORDATA  PortDimensions=2  SampleTime=3/120
  wires:
  SELF_Demux/1(x [m]) -> To Workspace/1, CC_x/1
  STATE_CyclingCyclist2_1_rc/1 -> STATE_CyclingCyclist2_1_bus/1
  STATE_CyclingCyclist2_1/1(StateBus) -> STATE_CyclingCyclist2_1_rc/1, Animation/1(In1)
  Animation/1(Out1) -> ANIM_CyclingCyclist2_1/1
  SELF_CyclingCyclist2_1/1 -> SELF_Demux/1(SELF)
  Trajectories/1(State) -> STATE_CyclingCyclist2_1/1(State)
  SELF_Demux/2(y [m]) -> To Workspace1/1, CC_y/1
  SELF_Demux/3(z [m]) -> Terminator_2/1
  SELF_Demux/4(rotx [deg]) -> Terminator_3/1
  SELF_Demux/5(roty [deg]) -> Terminator_4/1
  SELF_Demux/6(rotz [deg]) -> Terminator_5/1
  SELF_Demux/7(GPS lat [deg]) -> Terminator_6/1
  SELF_Demux/8(GPS long [deg]) -> Terminator_7/1
  SELF_Demux/9(GPS alt [m]) -> Terminator_8/1
  SELF_Demux/10(velocity [m/s]) -> Terminator_9/1
  SELF_Demux/11(heading [deg]) -> Terminator_10/1
  SELF_Demux/12(yaw rate [deg/s]) -> Terminator_11/1
  Ground_1/1 -> Scope3/1

== system Experiment_0309_cs_old/ObjectCameraSensor_1 ==
  Sensor : S-Function  FunctionName=sfun_OCS  Parameters=sensorID, detectableObjects, dataWidth, dataHeight, channelsPerImage, timestep  SFunctionDeploymentMode=off  EnableBusSupport=off  mask(PreScan Source Block: Object Camera Sensor){sensorID=439, detectableObjects=7, dataWidth=240, dataHeight=960, channelsPerImage=3, timestep=1/40}
      mask prompts: sensorID "Sensor ID"; detectableObjects "Max detectable objects:"; dataWidth "Data width"; dataHeight "Data Height"; channelsPerImage "Channels per image"; timestep "MATLAB timestep:"
      mask help: The Object Camera Sensor provides information on objects locations.
      mask Help: eval('openHelp(2401)')
      mask Display: image(imread('ObjectCameraSensorSL.png'))
  ObjectCameraSensor_1 : Outport  Tag=outport/ObjectCamera/data  OutDataTypeStr=Bus: PRESCAN_OCS_MESSAGE  PortDimensions=7  SampleTime=1/40
  ObjectCameraSensor_1_Image : Outport  Tag=outport/ObjectCamera/image  Port=2  OutDataTypeStr=uint8  SampleTime=1/40
  wires:
  Sensor/1 -> ObjectCameraSensor_1/1
  Sensor/2 -> ObjectCameraSensor_1_Image/1

== system Experiment_0309_cs_old/PreScanTerminator ==
  Terminator : Terminator
  sfun_Terminator : S-Function  FunctionName=sfun_Terminator  Parameters=SampleTime  SFunctionDeploymentMode=off  EnableBusSupport=off  mask(Legacy Function){SFunctionSpec=void prescan_terminator_outputFcn(void ** work1, PRESCAN_TERMINATORDATA y1[1]), SampleTime=TimeStep, ShowSpec=on}
      mask prompts: SampleTime "Sample time (-1 for inherited):"; ShowSpec "Display function specification"
      mask help:
      | This block allows you to call the legacy functions specified by the following Legacy Code Tool definition:
      | def.SFunctionName = 'sfun_Terminator';
      | def.OutputFcnSpec = 'void prescan_terminator_outputFcn(void ** work1, PRESCAN_TERMINATORDATA y1[1])';
      | def.StartFcnSpec = 'void prescan_terminator_startFcn(void ** work1)';
      | def.TerminateFcnSpec = 'void prescan_terminator_terminateFcn(void ** work1)';
      | def.HeaderFiles = {'prescan_terminator_data.h'};
      | def.HostLibFiles = {'sensorinterfaced.lib'};
      | def.IncPaths = {'src', 'C:\prescandev\vislibrary\vis\..\pimp\include\sensors\InterfaceRTW'};
      | def.SrcPaths = {'src'};
      | def.LibPaths = {'C:\\prescandev\\vislibrary_build\lib'};
      | def.SampleTime = 'parameterized';
      | def.Options.language = 'C';
      mask Help: <p>This block was generated automatically by the Legacy Code Tool. For detailed help on this tool, call<a href="matlab:legacy_code('help')"> legacy_code('help')</a>.</p>
      mask Callback ShowSpec:
      | if strcmp(get_param(gcbh, 'ShowSpec'), 'on')
      |   set_param(gcbh, 'MaskDisplay', sprintf('fprintf(''%s'');', get_param(gcbh, 'SFunctionSpec')));
      | else
      |   set_param(gcbh, 'MaskDisplay', sprintf('fprintf(''%s'');', get_param(gcbh, 'FunctionName')));
      | end
      mask Display: fprintf('void prescan_terminator_outputFcn(void ** work1, PRESCAN_TERMINATORDATA y1[1])');
  wires:
  sfun_Terminator/1 -> Terminator/1

== system Experiment_0309_cs_old/SELF_BMW_X5_SUV_1 ==
  Sensor : S-Function  FunctionName=sfun_SelfSensor  Parameters=UniqueID, TimeStep  SFunctionDeploymentMode=off  EnableBusSupport=off  mask(PreScan Source Block: SELF){UniqueID=266, TimeStep=3/120}
      mask prompts: UniqueID "Auto-Assigned: Unique ID"; TimeStep "Auto-Assigned: Upload Period [s]"
      mask help:
      | The SELF port shows (state) information of the actor itself. The outputs are position in the experiment's axis system and the GPS coordinates, and the object's absolute velocity and compass heading.
      |
      | For more information, please click Help.
      mask Help: eval('openHelp(462)')
      mask Display: image(imread('GPS.png'))
  SELF_BMW_X5_SUV_1 : Outport  Tag=outport/SelfPort  OutDataTypeStr=Bus: PRESCAN_SELFSENSORDATA  PortDimensions=1  SampleTime=3/120
  wires:
  Sensor/1 -> SELF_BMW_X5_SUV_1/1

== system Experiment_0309_cs_old/SELF_CyclingCyclist2_1 ==
  Sensor : S-Function  FunctionName=sfun_SelfSensor  Parameters=UniqueID, TimeStep  SFunctionDeploymentMode=off  EnableBusSupport=off  mask(PreScan Source Block: SELF){UniqueID=309, TimeStep=3/120}
      mask prompts: UniqueID "Auto-Assigned: Unique ID"; TimeStep "Auto-Assigned: Upload Period [s]"
      mask help:
      | The SELF port shows (state) information of the actor itself. The outputs are position in the experiment's axis system and the GPS coordinates, and the object's absolute velocity and compass heading.
      |
      | For more information, please click Help.
      mask Help: eval('openHelp(462)')
      mask Display: image(imread('GPS.png'))
  SELF_CyclingCyclist2_1 : Outport  Tag=outport/SelfPort  OutDataTypeStr=Bus: PRESCAN_SELFSENSORDATA  PortDimensions=1  SampleTime=3/120
  wires:
  Sensor/1 -> SELF_CyclingCyclist2_1/1

== system Experiment_0309_cs_old/STATE_BMW_X5_SUV_1_bus ==
  STATE_BMW_X5_SUV_1_bus : Inport  Tag=inport/StatePort  OutDataTypeStr=Bus: PRESCAN_STATEACTUATORDATA  PortDimensions=1  SampleTime=3/120  BusOutputAsStruct=on
  Actuator : S-Function  FunctionName=sfun_StateActuator  Parameters=UniqueID, TimeStep  SFunctionDeploymentMode=off  EnableBusSupport=off  mask(PreScan Sink Block: State){UniqueID=266, TimeStep=3/120}
      mask prompts: UniqueID "Auto-Assigned: Unique ID"; TimeStep "Auto-Assigned: Upload Period [s]"
      mask help:
      | The Actor State contains a vector signal of size (9x1), containing the following signals:
      |
      | -  Position    	(x,y,z)             	[m]
      | -  Velocity    	(vx,vy,vz)         	[m/s]
      | -  Angles       	(Roll, Pitch, Yaw)	[rad]
      |
      | The Actor state is defined in the global axis system.
      | The state is superponed on the Initial position defined in the GUI.
      |
      | For more information, please click Help.
      mask Help: eval('openHelp(222)')
      mask Display: image(imread('State.png'))
  wires:
  STATE_BMW_X5_SUV_1_bus/1 -> Actuator/1

== system Experiment_0309_cs_old/STATE_CyclingCyclist2_1_bus ==
  STATE_CyclingCyclist2_1_bus : Inport  Tag=inport/StatePort  OutDataTypeStr=Bus: PRESCAN_STATEACTUATORDATA  PortDimensions=1  SampleTime=3/120  BusOutputAsStruct=on
  Actuator : S-Function  FunctionName=sfun_StateActuator  Parameters=UniqueID, TimeStep  SFunctionDeploymentMode=off  EnableBusSupport=off  mask(PreScan Sink Block: State){UniqueID=309, TimeStep=3/120}
      mask prompts: UniqueID "Auto-Assigned: Unique ID"; TimeStep "Auto-Assigned: Upload Period [s]"
      mask help:
      | The Actor State contains a vector signal of size (9x1), containing the following signals:
      |
      | -  Position    	(x,y,z)             	[m]
      | -  Velocity    	(vx,vy,vz)         	[m/s]
      | -  Angles       	(Roll, Pitch, Yaw)	[rad]
      |
      | The Actor state is defined in the global axis system.
      | The state is superponed on the Initial position defined in the GUI.
      |
      | For more information, please click Help.
      mask Help: eval('openHelp(222)')
      mask Display: image(imread('State.png'))
  wires:
  STATE_CyclingCyclist2_1_bus/1 -> Actuator/1

== system Experiment_0309_cs_old/Synchronizer ==
  Bus Selector1 : BusSelector  OutputSignals=FederateStopped
  Stop Simulation : Stop
  sfun_Synchronizer : S-Function  FunctionName=sfun_Synchronizer  Parameters=SampleTime  SFunctionDeploymentMode=off  EnableBusSupport=off  mask(Legacy Function){SFunctionSpec=void prescan_synchronizer_outputFcn(void ** work1, PRESCAN_SYNCHRONIZEDATA y1[1]), SampleTime=TimeStep, ShowSpec=on}
      mask prompts: SampleTime "Sample time (-1 for inherited):"; ShowSpec "Display function specification"
      mask help:
      | This block allows you to call the legacy functions specified by the following Legacy Code Tool definition:
      | def.SFunctionName = 'sfun_Synchronizer';
      | def.OutputFcnSpec = 'void prescan_synchronizer_outputFcn(void ** work1, PRESCAN_SYNCHRONIZEDATA y1[1])';
      | def.StartFcnSpec = 'void prescan_synchronizer_startFcn(void ** work1)';
      | def.TerminateFcnSpec = 'void prescan_synchronizer_terminateFcn(void ** work1)';
      | def.HeaderFiles = {'prescan_synchronizer_data.h'};
      | def.HostLibFiles = {'sensorinterfaced.lib'};
      | def.IncPaths = {'src', 'C:\prescandev\vislibrary\vis\..\pimp\include\sensors\InterfaceRTW'};
      | def.SrcPaths = {'src'};
      | def.LibPaths = {'C:\\prescandev\\vislibrary_build\lib'};
      | def.SampleTime = 'parameterized';
      | def.Options.language = 'C';
      mask Help: <p>This block was generated automatically by the Legacy Code Tool. For detailed help on this tool, call<a href="matlab:legacy_code('help')"> legacy_code('help')</a>.</p>
      mask Callback ShowSpec:
      | if strcmp(get_param(gcbh, 'ShowSpec'), 'on')
      |   set_param(gcbh, 'MaskDisplay', sprintf('fprintf(''%s'');', get_param(gcbh, 'SFunctionSpec')));
      | else
      |   set_param(gcbh, 'MaskDisplay', sprintf('fprintf(''%s'');', get_param(gcbh, 'FunctionName')));
      | end
      mask Display: fprintf('void prescan_synchronizer_outputFcn(void ** work1, PRESCAN_SYNCHRONIZEDATA y1[1])');
  wires:
  Bus Selector1/1 -> Stop Simulation/1  "<FederateStopped>"
  sfun_Synchronizer/1 -> Bus Selector1/1

== system Experiment_0309_cs_old/TrafficLightDoubleKorean_1 ==
  Ground_{1..6} (6 alike) : Ground
  VISUCasingLights_1_Mux : Subsystem  Tag=mux/VisuCasingLights  mask(PreScan User Interface: VisuTrafficLight){}
      mask help:
      | The VisuTrafficLight block provides a way to animate traffic lights: switch on and off individual lights.
      |
      | For more information, please click Help.
      mask Help: eval('openHelp(731)')
  VISUCasingLights_2_Mux : Subsystem  Tag=mux/VisuCasingLights  mask(PreScan User Interface: VisuTrafficLight){}
      mask help:
      | The VisuTrafficLight block provides a way to animate traffic lights: switch on and off individual lights.
      |
      | For more information, please click Help.
      mask Help: eval('openHelp(731)')
  VISUCasingLights_1_TrafficLightDoubleKorean_1 : Outport  Tag=outport/VisuCasingLights  SampleTime=3/120
  VISUCasingLights_2_TrafficLightDoubleKorean_1 : Outport  Tag=outport/VisuCasingLights  Port=2  SampleTime=3/120
  wires:
  VISUCasingLights_1_Mux/1(VISUCasingLights_1_TrafficLightDoubleKorean_1) -> VISUCasingLights_1_TrafficLightDoubleKorean_1/1
  VISUCasingLights_2_Mux/1(VISUCasingLights_2_TrafficLightDoubleKorean_1) -> VISUCasingLights_2_TrafficLightDoubleKorean_1/1
  Ground_1/1 -> VISUCasingLights_1_Mux/1(Green [-])
  Ground_2/1 -> VISUCasingLights_1_Mux/2(Orange [-])
  Ground_3/1 -> VISUCasingLights_1_Mux/3(Red [-])
  Ground_4/1 -> VISUCasingLights_2_Mux/1(Green [-])
  Ground_5/1 -> VISUCasingLights_2_Mux/2(Orange [-])
  Ground_6/1 -> VISUCasingLights_2_Mux/3(Red [-])
